simulink model "IMPexamplesim"  (R2018a)
settings: Solver=VariableStepAuto  StartTime=0.0  StopTime=20  RelTol=1e-3
values from neighbouring files (symbols this model uses):
  ref = 70*2*pi/60    (= 7.33038285838)    [IMPexample.m]    (also in IMPexample2.m; IMPexample3.m)
  Ts = 0.01    [IMPexample.m]    (also in IMPexample2.m)
libraries: cstblocks x4, simulink x1
settings Model: Creator=Tobias Scala  LastModifiedBy=Tobias Scala

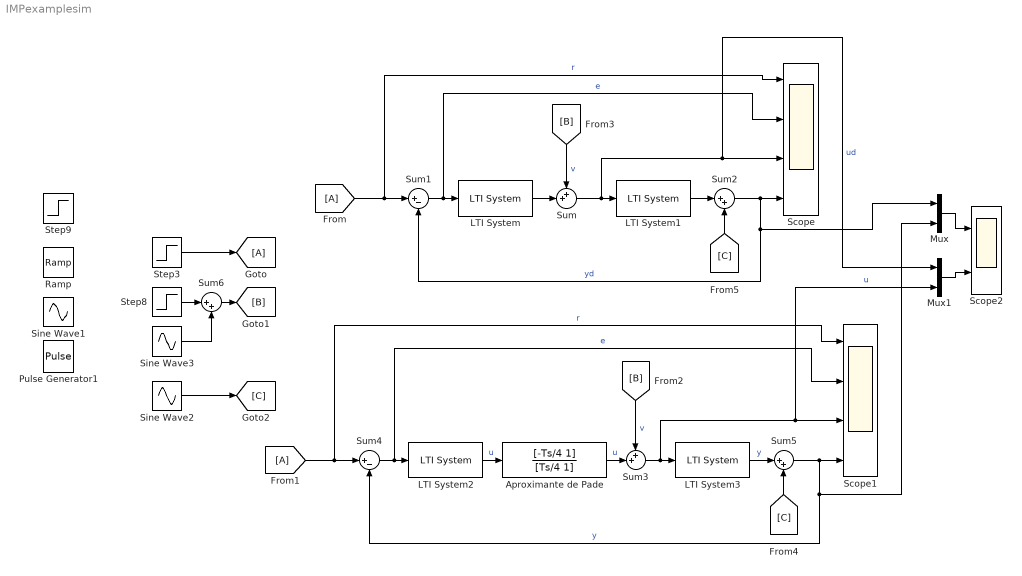
== system IMPexamplesim ==
  Aproximante de Pade : TransferFcn  Numerator=[-Ts/4 1]  Denominator=[Ts/4 1]
  LTI System : cstblocks/LTI System  sys=Cd  IC=[]
  LTI System1 : cstblocks/LTI System  sys=P  IC=[]
  LTI System2 : cstblocks/LTI System  sys=C  IC=[]
  LTI System3 : cstblocks/LTI System  sys=P  IC=[]
  Mux : Mux  Inputs=2
  Mux1 : Mux  Inputs=2
  Pulse Generator1 : DiscretePulseGenerator  PulseType=Time based  Period=10  PulseWidth=5
  Ramp : simulink/Sources/Ramp  slope=1  start=0  InitialOutput=0
  Scope : Scope  NumInputPorts=4
  Scope1 : Scope  NumInputPorts=4
  Scope2 : Scope  NumInputPorts=2
  Sine Wave1 : Sin  SampleTime=0
  Sine Wave2 : Sin  Amplitude=0  Frequency=100  SampleTime=0
  Sine Wave3 : Sin  Amplitude=2  Frequency=2*ref  SampleTime=0
  Step3 : Step  After=ref  SampleTime=0
  Step8 : Step  Time=10  After=2  SampleTime=0
  Step9 : Step  Time=15  After=0.5  SampleTime=0
  Sum : Sum  Inputs=++|
  Sum1 : Sum  Inputs=|+-
  Sum2 : Sum  Inputs=|++
  Sum3 : Sum  Inputs=++|
  Sum4 : Sum  Inputs=|+-
  Sum5 : Sum  Inputs=|++
  Sum6 : Sum  Inputs=|++
  wires:
  [B] -> Sum/1  "v"
  Sum1/1 -> LTI System/1, Scope/2  "e"
  [A] -> Sum1/1, Scope/1  "r"
  Sum2/1 -> Scope/4, Mux/1, Sum1/2  "yd"
  LTI System1/1 -> Sum2/1
  [C] -> Sum2/2
  Sum/1 -> Mux1/1, Scope/3, LTI System1/1  "ud"
  LTI System/1 -> Sum/2
  Sum3/1 -> Scope1/3, Mux1/2, LTI System3/1  "u"
  Sum5/1 -> Mux/2, Sum4/2, Scope1/4  "y"
  Sum4/1 -> LTI System2/1, Scope1/2  "e"
  LTI System3/1 -> Sum5/1  "y"
  [A] -> Sum4/1, Scope1/1  "r"
  [B] -> Sum3/1  "v"
  [C] -> Sum5/2
  LTI System2/1 -> Aproximante de Pade/1  "u"
  Aproximante de Pade/1 -> Sum3/2  "u"
  Step3/1 -> [A]
  Sine Wave2/1 -> [C]
  Mux/1 -> Scope2/1
  Mux1/1 -> Scope2/2
  Step8/1 -> Sum6/1
  Sum6/1 -> [B]
  Sine Wave3/1 -> Sum6/2
